simulink library "sm_car_scene_mcity"  (R2026a)
settings: Solver=VariableStepAuto
undefined symbols (not defined in the file or in its folder): Scene
libraries: Scene_Utilities x2
Description:
  | Scene of Simscape Vehicle Templates Library
  | 
  | Copyright 2018-2026 The MathWorks, Inc.
settings Model: Creator=smiller  LastModifiedBy=smiller

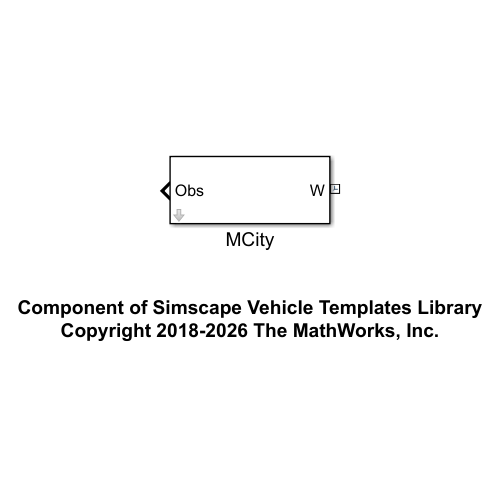
[thumbnail: Simulink's stored preview of the top-level diagram]
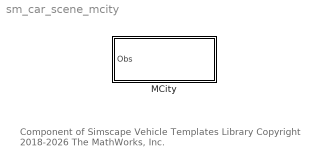
== system sm_car_scene_mcity ==
  note: Component of Simscape Vehicle Templates Library
      | Copyright 2018-2026 The MathWorks, Inc.
  MCity : Subsystem  mask{geometry=Scene.Pikes_Peak.Geometry}
      mask prompts: geometry "Geometry (structure)"

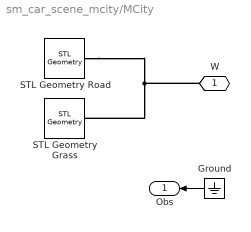
== system sm_car_scene_mcity/MCity ==
  Ground : Ground
  STL Geometry Grass : Scene_Utilities/STL Geometry  stl_file=geometry.grass.filename  stl_units=geometry.grass.fileunits  stl_clr=geometry.grass.clr  stl_opc=geometry.grass.opc  stl_x=geometry.grass.x  stl_y=geometry.grass.y  stl_z=geometry.grass.z  stl_yaw=geometry.grass.yaw  stl_pitch=geometry.grass.pitch  stl_roll=geometry.grass.roll
  STL Geometry Road : Scene_Utilities/STL Geometry  stl_file=geometry.filename  stl_units=geometry.fileunits  stl_clr=geometry.clr  stl_opc=geometry.opc  stl_x=geometry.x  stl_y=geometry.y  stl_z=geometry.z  stl_yaw=geometry.yaw  stl_pitch=geometry.pitch  stl_roll=geometry.roll
  W : PMIOPort  Side=Left
  Obs : Outport  VectorParamsAs1DForOutWhenUnconnected=off
  wires:
  Ground/1 -> Obs/1
  connections:
  STL Geometry Road/RConn1 -- STL Geometry Grass/RConn1 -- W/RConn1
